simulink model "Regulateurs"  (R2018b)
settings: Solver=VariableStepAuto  StartTime=0.0  StopTime=10  MaxStep=1e-3  RelTol=1e-3
values from neighbouring files (symbols this model uses):
  Cn = 643    [MAS23_init.m]
  Imr_refn = Frdn_max/Msr    [MAS23_init.m]
  J = 1.92    [MAS23_init.m]
  k = f    (= 0.0131717538735)    [MAS23_init.m]
  Kc = 1.6*3*to_c/sigma/Ts/(P*Msr^2/Lr*Imr_refn/Rs)    [MAS23_init.m]
  Kc1 = 0.28    [MAS23_init.m]
  Kf = 0.02*3/Tr    [MAS23_init.m]
  Kf1 = 0.3*3/Tr    [MAS23_init.m]
  Kv = 3    [MAS23_init.m]
  Lr = Lrr-Mr    [MAS23_init.m]
  Ls = Lss-Ms    [MAS23_init.m]
  Msr = 3/2*Msri    [MAS23_init.m]
  P = 1    [MAS23_init.m]
  Rs = Rp2    [MAS23_init.m]
  sigma = 1-Msr^2/Ls/Lr    [MAS23_init.m]
  TcBF = 0.0454/3    (= 0.0151333333333)    [MAS23_init.m]
  TfBF = 0.755/3    (= 0.251666666667)    [MAS23_init.m]
  to1_c = 1/(-poleC1)    [MAS23_init.m]
  to_c = 0.0055    [MAS23_init.m]
  to_f = 1/(-poleF(2))    [MAS23_init.m]
  to_v = J/k    (= 145.766465001)    [MAS23_init.m]
  Tr = Lr/Rr    [MAS23_init.m]
  Ts = Ls/Rs    [MAS23_init.m]
  Wb = 2*pi*freq    (= 314.159265359)    [MAS23_init.m]
settings Model: Creator=Louis  LastModifiedBy=jras
settings DataIOCC: SaveTime=off

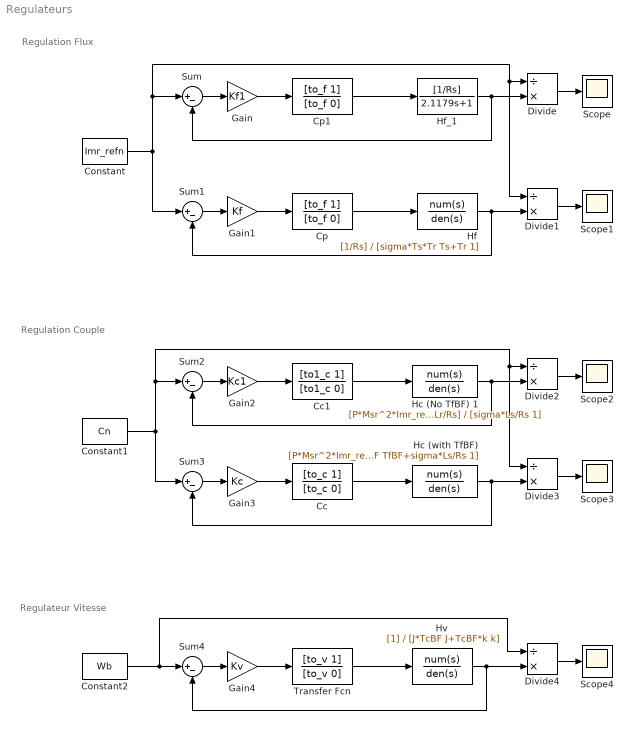
== system Regulateurs ==
  note: Regulateur Vitesse
  note: Regulation Couple
  note: Regulation Flux
  Cc : TransferFcn  Numerator=[to_c 1]  Denominator=[to_c 0]
  Cc1 : TransferFcn  Numerator=[to1_c 1]  Denominator=[to1_c 0]
  Constant : Constant  Value=Imr_refn
  Constant1 : Constant  Value=Cn
  Constant2 : Constant  Value=Wb
  Cp : TransferFcn  Numerator=[to_f 1]  Denominator=[to_f 0]
  Cp1 : TransferFcn  Numerator=[to_f 1]  Denominator=[to_f 0]
  Divide{,1..4} (5 alike) : Product  Inputs=/*
  Gain : Gain  Gain=Kf1
  Gain1 : Gain  Gain=Kf
  Gain2 : Gain  Gain=Kc1
  Gain3 : Gain  Gain=Kc
  Gain4 : Gain  Gain=Kv
  Hc (No TfBF) 1 : TransferFcn  Numerator=[P*Msr^2*Imr_refn/Lr/Rs]  Denominator=[sigma*Ls/Rs 1]
  Hc (with TfBF) : TransferFcn  Numerator=[P*Msr^2*Imr_refn/Lr/Rs]  Denominator=[sigma*Ls/Rs*TfBF TfBF+sigma*Ls/Rs 1]
  Hf : TransferFcn  Numerator=[1/Rs]  Denominator=[sigma*Ts*Tr Ts+Tr 1]
  Hf_1 : TransferFcn  Numerator=[1/Rs]  Denominator=[2.1179 1]
  Hv : TransferFcn  Denominator=[J*TcBF J+TcBF*k k]
  Scope{,1..4} (5 alike) : Scope
  Sum{,1..4} (5 alike) : Sum  Inputs=|+-
  Transfer Fcn : TransferFcn  Numerator=[to_v 1]  Denominator=[to_v 0]
  wires:
  Cp1/1 -> Hf_1/1
  Cp/1 -> Hf/1
  Gain/1 -> Cp1/1
  Gain1/1 -> Cp/1
  Sum/1 -> Gain/1
  Constant/1 -> Sum1/1, Divide/1, Divide1/1, Sum/1
  Sum1/1 -> Gain1/1
  Hf_1/1 -> Divide/2, Sum/2
  Hf/1 -> Divide1/2, Sum1/2
  Divide/1 -> Scope/1
  Divide1/1 -> Scope1/1
  Cc1/1 -> Hc (No TfBF) 1/1
  Cc/1 -> Hc (with TfBF)/1
  Gain2/1 -> Cc1/1
  Gain3/1 -> Cc/1
  Sum2/1 -> Gain2/1
  Hc (No TfBF) 1/1 -> Divide2/2, Sum2/2
  Sum3/1 -> Gain3/1
  Hc (with TfBF)/1 -> Divide3/2, Sum3/2
  Constant1/1 -> Sum3/1, Sum2/1, Divide3/1, Divide2/1
  Divide2/1 -> Scope2/1
  Divide3/1 -> Scope3/1
  Transfer Fcn/1 -> Hv/1
  Gain4/1 -> Transfer Fcn/1
  Sum4/1 -> Gain4/1
  Hv/1 -> Divide4/2, Sum4/2
  Constant2/1 -> Divide4/1, Sum4/1
  Divide4/1 -> Scope4/1
